simulink library "INT_PTSSE_SetData"  (R2016b)
settings: Solver=VariableStepAuto  StartTime=0.0  StopTime=10.0  RelTol=1e-3
settings Model: Creator=Wollf  LastModifiedBy=Wollf

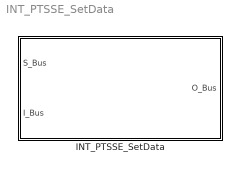
== system INT_PTSSE_SetData ==
  INT_PTSSE_SetData : Subsystem

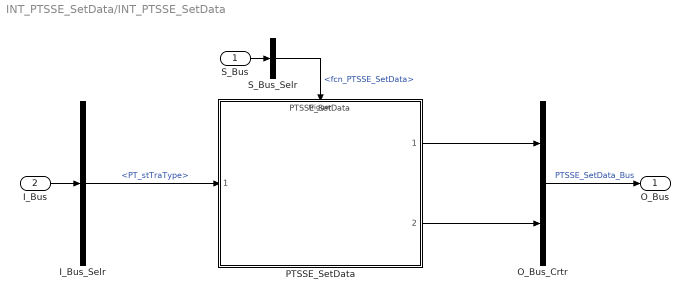
== system INT_PTSSE_SetData/INT_PTSSE_SetData ==
  S_Bus : Inport
  I_Bus : Inport  Port=2
  I_Bus_Selr : BusSelector  OutputSignals=PT_stTraType
  O_Bus_Crtr : BusCreator  Inputs=2
  PTSSE_SetData : ModelReference  ModelNameDialog=PTSSE_SetData  ModelReferenceVersion=1.1  TriggerPortName=function  TriggerPortTriggerType=function-call  TriggerPortStatesWhenEnabling=held
  S_Bus_Selr : BusSelector  OutputSignals=fcn_PTSSE_SetData
  O_Bus : Outport
  wires:
  S_Bus_Selr/1 -> PTSSE_SetData/Trigger  "<fcn_PTSSE_SetData>"
  S_Bus/1 -> S_Bus_Selr/1
  I_Bus/1 -> I_Bus_Selr/1
  I_Bus_Selr/1 -> PTSSE_SetData/1  "<PT_stTraType>"
  O_Bus_Crtr/1 -> O_Bus/1  "PTSSE_SetData_Bus"
  PTSSE_SetData/1 -> O_Bus_Crtr/1
  PTSSE_SetData/2 -> O_Bus_Crtr/2
